simulink model "adaptive_using_lyapunov"  (R2015b)
settings: Solver=VariableStepAuto  StartTime=0.0  StopTime=100  RelTol=1e-3
settings Model: Creator=uchiha  LastModifiedBy=uchiha

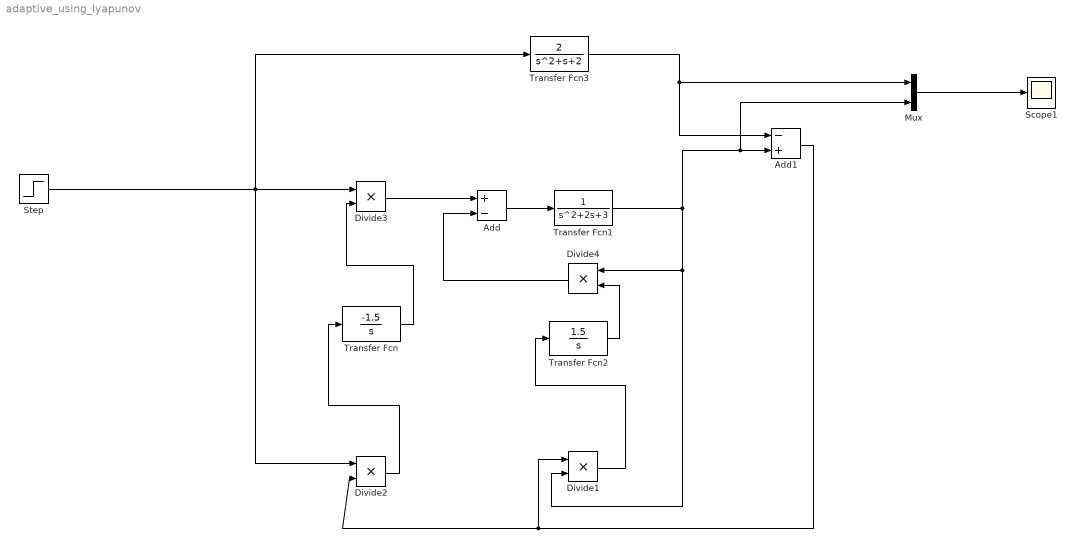
== system adaptive_using_lyapunov ==
  Add : Sum  Inputs=+-
  Add1 : Sum  Inputs=-+
  Divide{1..4} (4 alike) : Product  Inputs=**
  Mux : Mux  Inputs=2
  Scope1 : Scope
  Step : Step  SampleTime=0
  Transfer Fcn : TransferFcn  Numerator=[-1.5]  Denominator=[1 0]
  Transfer Fcn1 : TransferFcn  Denominator=[1 2 3]
  Transfer Fcn2 : TransferFcn  Numerator=[1.5]  Denominator=[1 0]
  Transfer Fcn3 : TransferFcn  Numerator=[2]  Denominator=[1 1 2]
  wires:
  Transfer Fcn/1 -> Divide3/2
  Divide2/1 -> Transfer Fcn/1
  Divide3/1 -> Add/1
  Add/1 -> Transfer Fcn1/1
  Transfer Fcn1/1 -> Divide1/2, Divide4/1, Mux/2, Add1/2
  Step/1 -> Transfer Fcn3/1, Divide2/1, Divide3/1
  Add1/1 -> Divide2/2, Divide1/1
  Divide1/1 -> Transfer Fcn2/1
  Transfer Fcn2/1 -> Divide4/2
  Divide4/1 -> Add/2
  Mux/1 -> Scope1/1
  Transfer Fcn3/1 -> Mux/1, Add1/1
